simulink model "IM_Model"  (R2018a)
settings: Solver=ode5  StartTime=0.0  StopTime=1  FixedStep=5e-6  RelTol=1e-3  EnableMultiTasking=on
InitFcn:
  | clc;
  | clear all;
  | % Parameters of a induction machine.
  | Vs=400; %Stator voltage
  | Rs=0.12; %Stator resistance
  | Rr=0.02; %Rotor resistance
  | Lls=0.0001; %Stator inductance
  | Llr=0.0001; %Rotor inductance
  | Lm=0.01;
  | P=2; %Number of Poles
  | Wg=2*pi*50;
  | s=0.02; % slip
  | Wr=(1-s)*Wg;
libraries: powerlib_meascontrol x1
settings Model: Creator=sa00g_000  LastModifiedBy=ShahRukh
settings DataIOCC: LimitDataPoints=on
settings OptimizationCC: LifeSpan=inf
settings DebuggingCC: AllowSymbolicDim=off  SFUnexpectedBacktrackingDiag=warning  SFNoUnconditionalDefaultTransitionDiag=warning  SFExecutionAtInitializationDiag=none
settings ModelReferenceCC: PropagateSignalLabelsOutOfModel=off
settings CodeAppCC: StateflowObjectComments=on
settings GRTTargetCC: TargetLangStandard=C89/C90 (ANSI)
settings ConfigComp: CovMetricSettings=dw  CovHtmlReporting=on  CovSaveCumulativeToWorkspaceVar=on  CovSaveSingleToWorkspaceVar=on  CovExternalEMLEnable=off

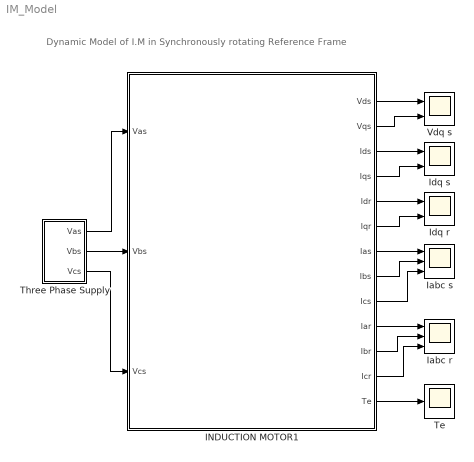
== system IM_Model ==
  note: Dynamic Model of I.M in Synchronously rotating Reference Frame
  " INDUCTION MOTOR1" : Subsystem
  Iabc r : Scope  NumInputPorts=3
  Iabc s : Scope  NumInputPorts=3
  Idq r : Scope  NumInputPorts=2
  Idq s : Scope  NumInputPorts=2
  Te : Scope
  Three Phase Supply : Subsystem
  Vdq s : Scope  NumInputPorts=2
  wires:
  " INDUCTION MOTOR1"/12(Icr) -> Iabc r/3
  " INDUCTION MOTOR1"/13(Te) -> Te/1
  " INDUCTION MOTOR1"/7(Ias) -> Iabc s/1
  " INDUCTION MOTOR1"/1(Vds) -> Vdq s/1
  " INDUCTION MOTOR1"/11(Ibr) -> Iabc r/2
  " INDUCTION MOTOR1"/8(Ibs) -> Iabc s/2
  " INDUCTION MOTOR1"/10(Iar) -> Iabc r/1
  " INDUCTION MOTOR1"/9(Ics) -> Iabc s/3
  " INDUCTION MOTOR1"/2(Vqs) -> Vdq s/2
  " INDUCTION MOTOR1"/5(Idr) -> Idq r/1
  " INDUCTION MOTOR1"/3(Ids) -> Idq s/1
  " INDUCTION MOTOR1"/4(Iqs) -> Idq s/2
  Three Phase Supply/1(Vas) -> " INDUCTION MOTOR1"/1(Vas)
  Three Phase Supply/2(Vbs) -> " INDUCTION MOTOR1"/2(Vbs)
  Three Phase Supply/3(Vcs) -> " INDUCTION MOTOR1"/3(Vcs)
  " INDUCTION MOTOR1"/6(Iqr) -> Idq r/2

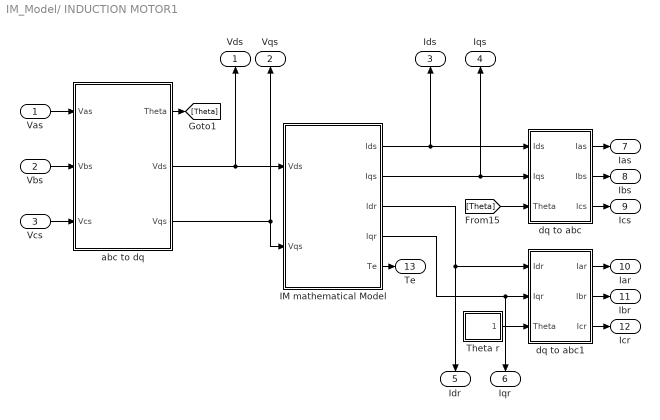
== system IM_Model/ INDUCTION MOTOR1 ==
  Vas : Inport
  Vbs : Inport  Port=2
  Vcs : Inport  Port=3
  IM mathematical Model : Subsystem
  Theta r : Subsystem
  abc to dq : Subsystem
  dq to abc : Subsystem
  dq to abc1 : Subsystem
  Vds : Outport
  Vqs : Outport  Port=2
  Ids : Outport  Port=3
  Iqs : Outport  Port=4
  Idr : Outport  Port=5
  Iqr : Outport  Port=6
  Ias : Outport  Port=7
  Ibs : Outport  Port=8
  Ics : Outport  Port=9
  Iar : Outport  Port=10
  Ibr : Outport  Port=11
  Icr : Outport  Port=12
  Te : Outport  Port=13
  wires:
  IM mathematical Model/1(Ids) -> Ids/1, dq to abc/1(Ids)
  IM mathematical Model/2(Iqs) -> Iqs/1, dq to abc/2(Iqs)
  abc to dq/2(Vds) -> Vds/1, IM mathematical Model/1(Vds)
  abc to dq/3(Vqs) -> IM mathematical Model/2(Vqs), Vqs/1
  Vas/1 -> abc to dq/1(Vas)
  IM mathematical Model/5(Te) -> Te/1
  Vcs/1 -> abc to dq/3(Vcs)
  Vbs/1 -> abc to dq/2(Vbs)
  abc to dq/1(Theta) -> [Theta]
  [Theta] -> dq to abc/3(Theta)
  IM mathematical Model/3(Idr) -> Idr/1, dq to abc1/1(Idr)
  IM mathematical Model/4(Iqr) -> Iqr/1, dq to abc1/2(Iqr)
  Theta r/1(Theta_r) -> dq to abc1/3(Theta)
  dq to abc/1(Ias) -> Ias/1
  dq to abc/2(Ibs) -> Ibs/1
  dq to abc/3(Ics) -> Ics/1
  dq to abc1/1(Iar) -> Iar/1
  dq to abc1/2(Ibr) -> Ibr/1
  dq to abc1/3(Icr) -> Icr/1

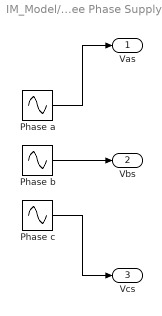
== system IM_Model/Three Phase Supply ==
  Phase a : Sin  Amplitude=Vs*sqrt(2)/sqrt(3)  Frequency=2*pi*50  SampleTime=0
  Phase b : Sin  Amplitude=Vs*sqrt(2)/sqrt(3)  Frequency=2*pi*50  Phase=-2*pi/3  SampleTime=0
  Phase c : Sin  Amplitude=Vs*sqrt(2)/sqrt(3)  Frequency=2*pi*50  Phase=2*pi/3  SampleTime=0
  Vas : Outport
  Vbs : Outport  Port=2
  Vcs : Outport  Port=3
  wires:
  Phase b/1 -> Vbs/1
  Phase a/1 -> Vas/1
  Phase c/1 -> Vcs/1

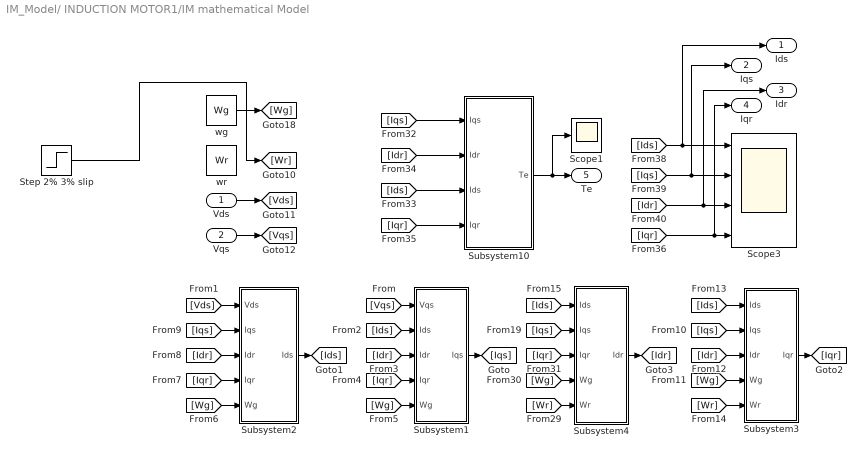
== system IM_Model/ INDUCTION MOTOR1/IM mathematical Model ==
  Vds : Inport
  Vqs : Inport  Port=2
  Scope1 : Scope
  Scope3 : Scope  NumInputPorts=4
  Step 2% 3% slip : Step  Time=0.5  Before=(1-0.02)*2*pi*50  After=(1-0.04)*2*pi*50  SampleTime=0
  Subsystem1 : Subsystem
  Subsystem10 : Subsystem
  Subsystem2 : Subsystem
  Subsystem3 : Subsystem
  Subsystem4 : Subsystem
  wg : Constant  Value=Wg
  wr : Constant  Value=Wr
  Ids : Outport
  Iqs : Outport  Port=2
  Idr : Outport  Port=3
  Iqr : Outport  Port=4
  Te : Outport  Port=5
  wires:
  wg/1 -> [Wg]
  Subsystem4/1(Idr) -> [Idr]
  [Iqs] -> Subsystem3/2(Iqs)
  [Wg] -> Subsystem1/5(Wg)
  [Ids] -> Subsystem3/1(Ids)
  [Iqr] -> Subsystem1/4(Iqr)
  [Idr] -> Subsystem3/3(Idr)
  [Wr] -> Subsystem3/5(Wr)
  [Vqs] -> Subsystem1/1(Vqs)
  Subsystem2/1(Ids) -> [Ids]
  Subsystem1/1(Iqs) -> [Iqs]
  [Ids] -> Subsystem10/3(Ids)
  [Iqs] -> Subsystem10/1(Iqs)
  [Idr] -> Subsystem10/2(Idr)
  [Ids] -> Subsystem1/2(Ids)
  [Ids] -> Scope3/1, Ids/1
  [Ids] -> Subsystem4/1(Ids)
  [Iqr] -> Subsystem4/3(Iqr)
  Subsystem3/1(Iqr) -> [Iqr]
  [Iqs] -> Subsystem4/2(Iqs)
  [Wg] -> Subsystem4/4(Wg)
  [Iqs] -> Scope3/2, Iqs/1
  [Wg] -> Subsystem3/4(Wg)
  [Iqr] -> Subsystem10/4(Iqr)
  [Wr] -> Subsystem4/5(Wr)
  [Idr] -> Subsystem1/3(Idr)
  Vqs/1 -> [Vqs]
  Vds/1 -> [Vds]
  [Vds] -> Subsystem2/1(Vds)
  [Iqs] -> Subsystem2/2(Iqs)
  [Idr] -> Subsystem2/3(Idr)
  [Iqr] -> Subsystem2/4(Iqr)
  [Wg] -> Subsystem2/5(Wg)
  [Iqr] -> Iqr/1, Scope3/4
  [Idr] -> Idr/1, Scope3/3
  Subsystem10/1(Te) -> Scope1/1, Te/1
  Step 2% 3% slip/1 -> [Wr]

== system IM_Model/ INDUCTION MOTOR1/Theta r ==
  Gain : Gain  Gain=pi
  Sawtooth Generator : powerlib_meascontrol/Pulse & Signal Generators/Sawtooth Generator  Freq=s*50  Phase=90  Ts=0
      settings: SourceProductName=Simscape Power Systems
  Theta_r : Outport
  wires:
  Sawtooth Generator/1 -> Gain/1
  Gain/1 -> Theta_r/1

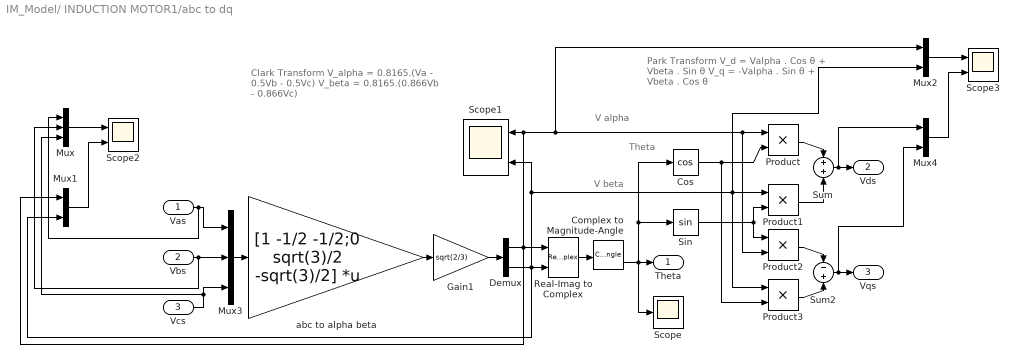
== system IM_Model/ INDUCTION MOTOR1/abc to dq ==
  note: V alpha
  note: Clark Transform
      | V_alpha = 0.8165.(Va - 0.5Vb - 0.5Vc)
      | V_beta = 0.8165.(0.866Vb - 0.866Vc)
  note: Park Transform
      | V_d = Valpha . Cos θ + Vbeta . Sin θ
      | V_q = -Valpha . Sin θ + Vbeta . Cos θ
  note: V beta
  note: Theta
  Vas : Inport
  Vbs : Inport  Port=2
  Vcs : Inport  Port=3
  Complex to Magnitude-Angle : ComplexToMagnitudeAngle
  Cos : Trigonometry  Operator=cos
  Demux : Demux  Outputs=2
  Gain1 : Gain  Gain=sqrt(2/3)
  Mux : Mux  Inputs=3
  Mux1 : Mux  Inputs=2
  Mux2 : Mux  Inputs=2
  Mux3 : Mux  Inputs=3
  Mux4 : Mux  Inputs=2
  Product{,1..3} (4 alike) : Product
  Real-Imag to Complex : RealImagToComplex
  Scope : Scope
  Scope1 : Scope  NumInputPorts=2
  Scope2 : Scope  NumInputPorts=2
  Scope3 : Scope  NumInputPorts=2
  "Sin " : Trigonometry
  Sum : Sum
  Sum2 : Sum  Inputs=-+
  abc to alpha beta : Gain  Gain=[1 -1/2 -1/2;0 sqrt(3)/2 -sqrt(3)/2]  Multiplication=Matrix(K*u)
  Theta : Outport
  Vds : Outport  Port=2
  Vqs : Outport  Port=3
  wires:
  Complex to Magnitude-Angle/2 -> "Sin "/1, Cos/1, Scope/1, Theta/1
  abc to alpha beta/1 -> Gain1/1
  Gain1/1 -> Demux/1
  Real-Imag to Complex/1 -> Complex to Magnitude-Angle/1
  Mux3/1 -> abc to alpha beta/1
  Vas/1 -> Mux/1, Mux3/1
  Vbs/1 -> Mux/2, Mux3/2
  Vcs/1 -> Mux3/3, Mux/3
  Product3/1 -> Sum2/2
  Demux/2 -> Product3/1, Product1/1, Mux2/2, Scope1/2, Mux1/2, Real-Imag to Complex/2
  Demux/1 -> Mux2/1, Product2/2, Product/1, Scope1/1, Mux1/1, Real-Imag to Complex/1
  Sum/1 -> Mux4/1, Vds/1
  Product/1 -> Sum/1
  "Sin "/1 -> Product2/1, Product1/2
  Cos/1 -> Product/2, Product3/2
  Sum2/1 -> Mux4/2, Vqs/1
  Product1/1 -> Sum/2
  Product2/1 -> Sum2/1
  Mux/1 -> Scope2/1
  Mux1/1 -> Scope2/2
  Mux2/1 -> Scope3/1
  Mux4/1 -> Scope3/2

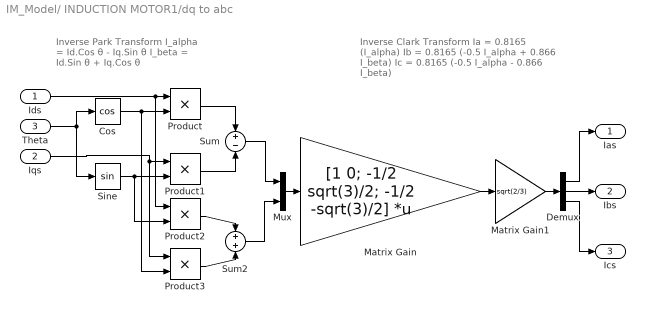
== system IM_Model/ INDUCTION MOTOR1/dq to abc ==
  note: Inverse Park Transform
      | I_alpha = Id.Cos θ - Iq.Sin θ
      | I_beta = Id.Sin θ + Iq.Cos θ
  note: Inverse Clark Transform
      | Ia = 0.8165 (I_alpha)
      | Ib = 0.8165 (-0.5 I_alpha + 0.866 I_beta)
      | Ic = 0.8165 (-0.5 I_alpha - 0.866 I_beta)
  Ids : Inport
  Iqs : Inport  Port=2
  Theta : Inport  Port=3
  Cos : Trigonometry  Operator=cos
  Demux : Demux  Outputs=3
  Matrix Gain : Gain  Gain=[1 0; -1/2 sqrt(3)/2; -1/2 -sqrt(3)/2]  Multiplication=Matrix(K*u)  SaturateOnIntegerOverflow=on  OutDataTypeStr=Inherit: Same as input  ParamDataTypeStr=Inherit: Same as input
  Matrix Gain1 : Gain  Gain=sqrt(2/3)  SaturateOnIntegerOverflow=on  OutDataTypeStr=Inherit: Same as input  ParamDataTypeStr=Inherit: Same as input
  Mux : Mux  Inputs=2
  Product{,1..3} (4 alike) : Product
  "Sine " : Trigonometry
  Sum : Sum  Inputs=+-
  Sum2 : Sum
  Ias : Outport
  Ibs : Outport  Port=2
  Ics : Outport  Port=3
  wires:
  Product3/1 -> Sum2/2
  Product2/1 -> Sum2/1
  Product1/1 -> Sum/2
  Product/1 -> Sum/1
  Cos/1 -> Product3/2, Product/2
  Ids/1 -> Product2/1, Product/1
  Iqs/1 -> Product3/1, Product1/1
  Theta/1 -> "Sine "/1, Cos/1
  "Sine "/1 -> Product2/2, Product1/2
  Matrix Gain1/1 -> Demux/1
  Demux/3 -> Ics/1
  Mux/1 -> Matrix Gain/1
  Matrix Gain/1 -> Matrix Gain1/1
  Sum2/1 -> Mux/2
  Demux/2 -> Ibs/1
  Demux/1 -> Ias/1
  Sum/1 -> Mux/1

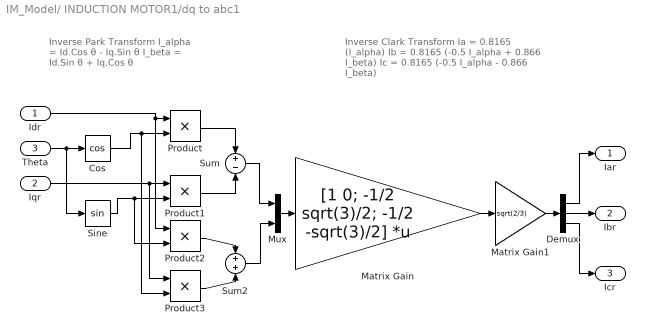
== system IM_Model/ INDUCTION MOTOR1/dq to abc1 ==
  note: Inverse Park Transform
      | I_alpha = Id.Cos θ - Iq.Sin θ
      | I_beta = Id.Sin θ + Iq.Cos θ
  note: Inverse Clark Transform
      | Ia = 0.8165 (I_alpha)
      | Ib = 0.8165 (-0.5 I_alpha + 0.866 I_beta)
      | Ic = 0.8165 (-0.5 I_alpha - 0.866 I_beta)
  Idr : Inport
  Iqr : Inport  Port=2
  Theta : Inport  Port=3
  Cos : Trigonometry  Operator=cos
  Demux : Demux  Outputs=3
  Matrix Gain : Gain  Gain=[1 0; -1/2 sqrt(3)/2; -1/2 -sqrt(3)/2]  Multiplication=Matrix(K*u)  SaturateOnIntegerOverflow=on  OutDataTypeStr=Inherit: Same as input  ParamDataTypeStr=Inherit: Same as input
  Matrix Gain1 : Gain  Gain=sqrt(2/3)  SaturateOnIntegerOverflow=on  OutDataTypeStr=Inherit: Same as input  ParamDataTypeStr=Inherit: Same as input
  Mux : Mux  Inputs=2
  Product{,1..3} (4 alike) : Product
  "Sine " : Trigonometry
  Sum : Sum  Inputs=+-
  Sum2 : Sum
  Iar : Outport
  Ibr : Outport  Port=2
  Icr : Outport  Port=3
  wires:
  Product3/1 -> Sum2/2
  Product2/1 -> Sum2/1
  Product1/1 -> Sum/2
  Product/1 -> Sum/1
  Cos/1 -> Product3/2, Product/2
  Idr/1 -> Product2/1, Product/1
  Iqr/1 -> Product3/1, Product1/1
  Theta/1 -> Cos/1, "Sine "/1
  "Sine "/1 -> Product2/2, Product1/2
  Demux/3 -> Icr/1
  Mux/1 -> Matrix Gain/1
  Matrix Gain1/1 -> Demux/1
  Demux/1 -> Iar/1
  Matrix Gain/1 -> Matrix Gain1/1
  Sum/1 -> Mux/1
  Demux/2 -> Ibr/1
  Sum2/1 -> Mux/2

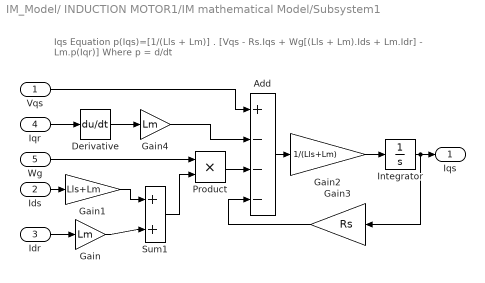
== system IM_Model/ INDUCTION MOTOR1/IM mathematical Model/Subsystem1 ==
  note: Iqs Equation
      | p(Iqs)=[1/(Lls + Lm)] . [Vqs - Rs.Iqs + Wg[(Lls + Lm).Ids + Lm.Idr] - Lm.p(Iqr)]
      | Where p = d/dt
  Vqs : Inport
  Ids : Inport  Port=2
  Idr : Inport  Port=3
  Iqr : Inport  Port=4
  Wg : Inport  Port=5
  Add : Sum  Inputs=+---
  Derivative : Derivative
  Gain : Gain  Gain=Lm
  Gain1 : Gain  Gain=Lls+Lm
  Gain2 : Gain  Gain=1/(Lls+Lm)
  Gain3 : Gain  Gain=Rs
  Gain4 : Gain  Gain=Lm
  Integrator : Integrator
  Product : Product
  Sum1 : Sum  Inputs=|++
  Iqs : Outport
  wires:
  Product/1 -> Add/3
  Wg/1 -> Product/1
  Gain4/1 -> Add/2
  Gain3/1 -> Add/4
  Derivative/1 -> Gain4/1
  Gain2/1 -> Integrator/1
  Vqs/1 -> Add/1
  Iqr/1 -> Derivative/1
  Add/1 -> Gain2/1
  Gain1/1 -> Sum1/1
  Ids/1 -> Gain1/1
  Sum1/1 -> Product/2
  Gain/1 -> Sum1/2
  Idr/1 -> Gain/1
  Integrator/1 -> Iqs/1, Gain3/1

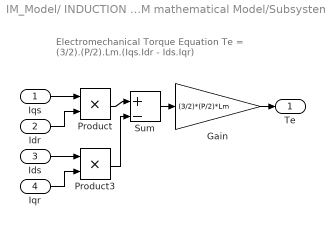
== system IM_Model/ INDUCTION MOTOR1/IM mathematical Model/Subsystem10 ==
  note: Electromechanical Torque Equation
      | Te = (3/2).(P/2).Lm.(Iqs.Idr - Ids.Iqr)
  Iqs : Inport
  Idr : Inport  Port=2
  Ids : Inport  Port=3
  Iqr : Inport  Port=4
  Gain : Gain  Gain=(3/2)*(P/2)*Lm
  Product : Product
  Product3 : Product
  Sum : Sum  Inputs=|+-
  Te : Outport
  wires:
  Product/1 -> Sum/1
  Sum/1 -> Gain/1
  Product3/1 -> Sum/2
  Gain/1 -> Te/1
  Iqs/1 -> Product/1
  Idr/1 -> Product/2
  Ids/1 -> Product3/1
  Iqr/1 -> Product3/2

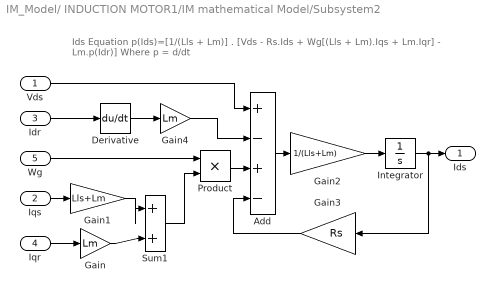
== system IM_Model/ INDUCTION MOTOR1/IM mathematical Model/Subsystem2 ==
  note: Ids Equation
      | p(Ids)=[1/(Lls + Lm)] . [Vds - Rs.Ids + Wg[(Lls + Lm).Iqs + Lm.Iqr] - Lm.p(Idr)]
      | Where p = d/dt
  Vds : Inport
  Iqs : Inport  Port=2
  Idr : Inport  Port=3
  Iqr : Inport  Port=4
  Wg : Inport  Port=5
  Add : Sum  Inputs=+-+-
  Derivative : Derivative
  Gain : Gain  Gain=Lm
  Gain1 : Gain  Gain=Lls+Lm
  Gain2 : Gain  Gain=1/(Lls+Lm)
  Gain3 : Gain  Gain=Rs
  Gain4 : Gain  Gain=Lm
  Integrator : Integrator
  Product : Product
  Sum1 : Sum  Inputs=|++
  Ids : Outport
  wires:
  Integrator/1 -> Gain3/1, Ids/1
  Iqr/1 -> Gain/1
  Gain/1 -> Sum1/2
  Sum1/1 -> Product/2
  Iqs/1 -> Gain1/1
  Gain1/1 -> Sum1/1
  Add/1 -> Gain2/1
  Idr/1 -> Derivative/1
  Vds/1 -> Add/1
  Gain2/1 -> Integrator/1
  Derivative/1 -> Gain4/1
  Gain3/1 -> Add/4
  Gain4/1 -> Add/2
  Wg/1 -> Product/1
  Product/1 -> Add/3

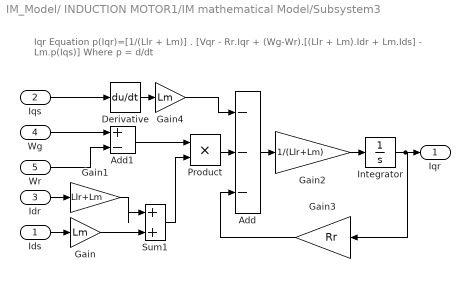
== system IM_Model/ INDUCTION MOTOR1/IM mathematical Model/Subsystem3 ==
  note: Iqr Equation
      | p(Iqr)=[1/(Llr + Lm)] . [Vqr - Rr.Iqr + (Wg-Wr).[(Llr + Lm).Idr + Lm.Ids] - Lm.p(Iqs)]
      | Where p = d/dt
  Ids : Inport
  Iqs : Inport  Port=2
  Idr : Inport  Port=3
  Wg : Inport  Port=4
  Wr : Inport  Port=5
  Add : Sum  Inputs=---
  Add1 : Sum  Inputs=+-
  Derivative : Derivative
  Gain : Gain  Gain=Lm
  Gain1 : Gain  Gain=Llr+Lm
  Gain2 : Gain  Gain=1/(Llr+Lm)
  Gain3 : Gain  Gain=Rr
  Gain4 : Gain  Gain=Lm
  Integrator : Integrator
  Product : Product
  Sum1 : Sum  Inputs=|++
  Iqr : Outport
  wires:
  Gain3/1 -> Add/3
  Derivative/1 -> Gain4/1
  Gain2/1 -> Integrator/1
  Iqs/1 -> Derivative/1
  Add/1 -> Gain2/1
  Gain1/1 -> Sum1/1
  Idr/1 -> Gain1/1
  Sum1/1 -> Product/2
  Gain/1 -> Sum1/2
  Ids/1 -> Gain/1
  Integrator/1 -> Gain3/1, Iqr/1
  Wg/1 -> Add1/1
  Add1/1 -> Product/1
  Wr/1 -> Add1/2
  Gain4/1 -> Add/1
  Product/1 -> Add/2

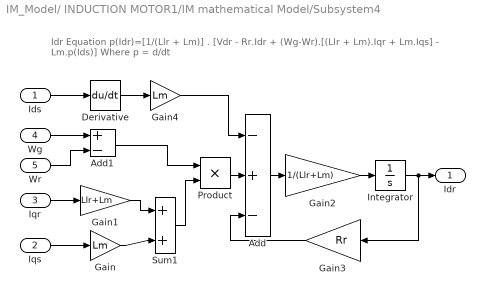
== system IM_Model/ INDUCTION MOTOR1/IM mathematical Model/Subsystem4 ==
  note: Idr Equation
      | p(Idr)=[1/(Llr + Lm)] . [Vdr - Rr.Idr + (Wg-Wr).[(Llr + Lm).Iqr + Lm.Iqs] - Lm.p(Ids)]
      | Where p = d/dt
  Ids : Inport
  Iqs : Inport  Port=2
  Iqr : Inport  Port=3
  Wg : Inport  Port=4
  Wr : Inport  Port=5
  Add : Sum  Inputs=-+-
  Add1 : Sum  Inputs=+-
  Derivative : Derivative
  Gain : Gain  Gain=Lm
  Gain1 : Gain  Gain=Llr+Lm
  Gain2 : Gain  Gain=1/(Llr+Lm)
  Gain3 : Gain  Gain=Rr
  Gain4 : Gain  Gain=Lm
  Integrator : Integrator
  Product : Product
  Sum1 : Sum  Inputs=|++
  Idr : Outport
  wires:
  Product/1 -> Add/2
  Gain4/1 -> Add/1
  Wr/1 -> Add1/2
  Add1/1 -> Product/1
  Wg/1 -> Add1/1
  Integrator/1 -> Gain3/1, Idr/1
  Iqs/1 -> Gain/1
  Gain/1 -> Sum1/2
  Sum1/1 -> Product/2
  Iqr/1 -> Gain1/1
  Gain1/1 -> Sum1/1
  Add/1 -> Gain2/1
  Ids/1 -> Derivative/1
  Gain2/1 -> Integrator/1
  Derivative/1 -> Gain4/1
  Gain3/1 -> Add/3
